simulink model "plant2016_cybership_non_adaptive"  (R2015b)
settings: Solver=VariableStepAuto  StartTime=0.0  StopTime=1000  RelTol=1e-3
libraries: simulink x4
settings Model: Creator=TordFO  LastModifiedBy=TordFO

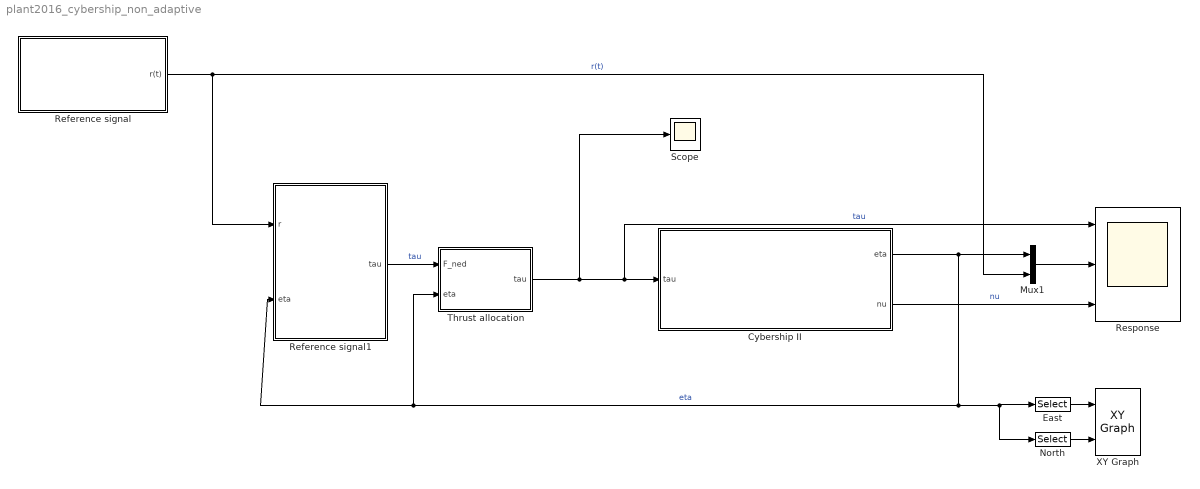
== system plant2016_cybership_non_adaptive ==
  Cybership II : Subsystem  mask{eta_0=[0;0;0]%[1;2;20*pi/180], nu_0=[0;0;0], first_order_waves_on_off=off, wind_on_off=on, surge_only=off}
      mask prompts: eta_0 "Position initial state"; nu_0 "Velocity initial state"; first_order_waves_on_off "First order wave disturbances"; wind_on_off "Wind loads"; surge_only "Only surge"
      mask Display: image('CybershipIII.jpg')
  East : Selector  InputPortWidth=3  IndexOptions=Index vector (dialog)  Indices=[2]  OutputSizes=1
  Mux1 : Mux  Inputs=2
  North : Selector  InputPortWidth=3  IndexOptions=Index vector (dialog)  Indices=[1]  OutputSizes=1
  Reference signal : Subsystem
  Reference signal1 : Subsystem  mask(SISO 3 DOF controller){surge_Kp=2.7, surge_Ki=0.1, surge_Kd=10, sway_Kp=2, sway_Ki=0.1, sway_Kd=10, yaw_Kp=2, yaw_Ki=0.3, yaw_Kd=2, surge_epsilon=0.01, sway_epsilon=0.01, yaw_epsilon=0.01}
      mask prompts: surge_Kp "Kp-gain"; surge_Ki "Ki-gain"; surge_Kd "Kd-gain"; sway_Kp "Kp-gain"; sway_Ki "Ki-gain"; sway_Kd "Kd-gain"; yaw_Kp "Kp-gain"; yaw_Ki "Ki-gain"; yaw_Kd "Kd-gain"; surge_epsilon "Surge epsilon"; sway_epsilon "Sway epsilon"; yaw_epsilon "Yaw epsilon"
      mask help: The masked subsystem is a 3 DOF controller for planear motion ship control. The controller replicates the structure of the self-tuning unfalsified PID controller, here with fixed gain to compare behaviour
      mask Help: Activate any combinations of the SISO controllers. Gains and epsolon values should be positive. Epsilon values are added derivative term in denominator to make controller biproper. Set gain values for activated controller other that zero (not required) to use the controller.
      mask Display: image('control_system.png')
  Response : Scope  NumInputPorts=3
  Scope : Scope
  Thrust allocation : Subsystem  mask(Thrust allocation block){surge_control_on_off=on, sway_control_on_off=on, yaw_control_on_off=on}
      mask prompts: surge_control_on_off "Surge Thrust on"; sway_control_on_off "Sway Thrust on"; yaw_control_on_off "Yaw Thrust on"
      mask help: Thrust allocation block. The block rotates the NED-force vector to the body frame where the ship is actuated in pure surge, sway and yaw. Any of the thrust direction can be enabeled/disabeled, but note that reference tracking is only possible for both surge and sway thrust enabeled.
  XY Graph : simulink/Sinks/XY Graph  xmin=-10  xmax=10  ymin=-10  ymax=10  st=-1
  wires:
  Reference signal/1(r(t)) -> Reference signal1/1(r), Mux1/2  "r(t)"
  Cybership II/2(nu) -> Response/3  "nu"
  Mux1/1 -> Response/2
  North/1 -> XY Graph/2
  East/1 -> XY Graph/1
  Cybership II/1(eta) -> Mux1/1, Reference signal1/2(eta), Thrust allocation/2(eta), North/1, East/1  "eta"
  Thrust allocation/1(tau) -> Scope/1, Cybership II/1(tau), Response/1  "tau"
  Reference signal1/1(tau) -> Thrust allocation/1(F_ned)  "tau"

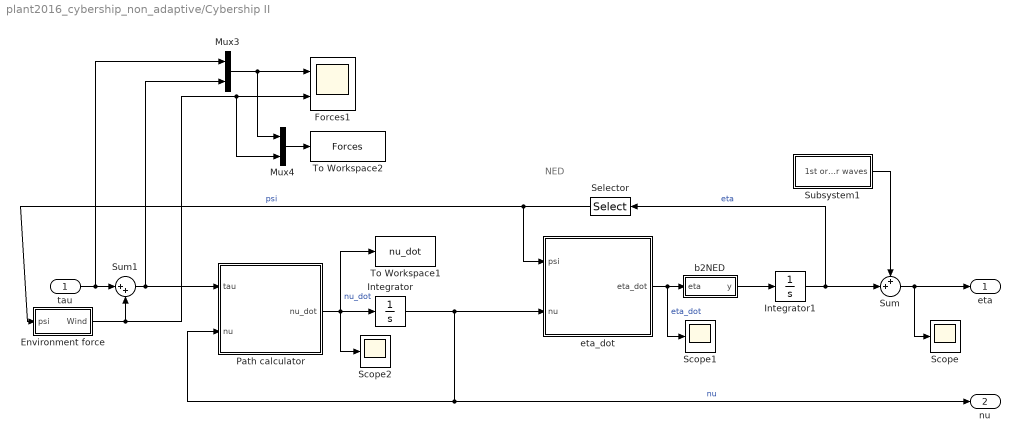
== system plant2016_cybership_non_adaptive/Cybership II ==
  note: NED
  tau : Inport
  Environment force : Subsystem
  Forces1 : Scope  NumInputPorts=2
  Integrator : Integrator  InitialCondition=nu_0
  Integrator1 : Integrator  InitialCondition=eta_0
  Mux3 : Mux  Inputs=2
  Mux4 : Mux  Inputs=2
  Path calculator : MATLAB Function  TreatAsAtomicUnit=on
  Scope : Scope
  Scope1 : Scope
  Scope2 : Scope
  Selector : Selector  InputPortWidth=3  IndexOptions=Index vector (dialog)  Indices=3  OutputSizes=1
  Subsystem1 : Subsystem
  Sum : Sum  Inputs=++|
  Sum1 : Sum  Inputs=|++
  To Workspace1 : ToWorkspace  VariableName=nu_dot  SaveFormat=Timeseries  SampleTime=-1
  To Workspace2 : ToWorkspace  VariableName=Forces  SaveFormat=Timeseries  SampleTime=-1
  b2NED : MATLAB Function  TreatAsAtomicUnit=on
  eta_dot : MATLAB Function  TreatAsAtomicUnit=on
  eta : Outport
  nu : Outport  Port=2
  wires:
  Sum1/1 -> Mux3/2, Path calculator/1(tau)
  eta_dot/1(eta_dot) -> Scope1/1, b2NED/1(eta)  "eta_dot"
  Path calculator/1(nu_dot) -> Scope2/1, To Workspace1/1, Integrator/1  "nu_dot"
  Integrator1/1 -> Sum/2, Selector/1  "eta"
  Integrator/1 -> nu/1, Path calculator/2(nu), eta_dot/2(nu)  "nu"
  Selector/1 -> eta_dot/1(psi), Environment force/1(psi)  "psi"
  b2NED/1(y) -> Integrator1/1
  Sum/1 -> Scope/1, eta/1
  Subsystem1/1(1st order waves) -> Sum/1
  tau/1 -> Mux3/1, Sum1/1
  Environment force/1(Wind) -> Forces1/2, Mux4/2, Sum1/2
  Mux3/1 -> Forces1/1, Mux4/1
  Mux4/1 -> To Workspace2/1

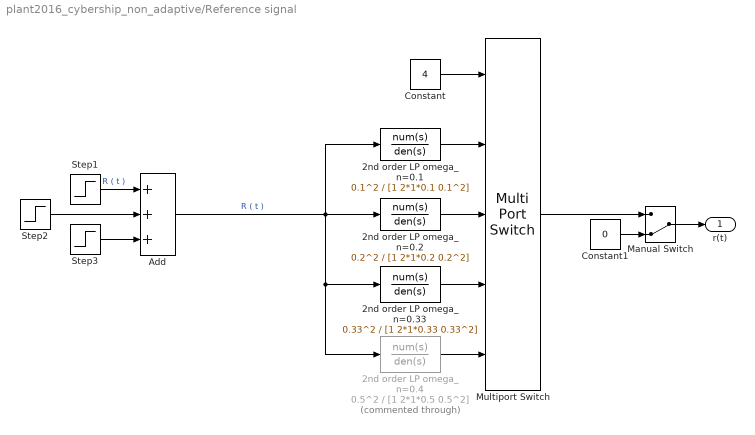
== system plant2016_cybership_non_adaptive/Reference signal ==
  2nd order LP omega_n=0.1 : TransferFcn  Numerator=0.1^2  Denominator=[1 2*1*0.1 0.1^2]
  2nd order LP omega_n=0.2 : TransferFcn  Numerator=0.2^2  Denominator=[1 2*1*0.2 0.2^2]
  2nd order LP omega_n=0.33 : TransferFcn  Numerator=0.33^2  Denominator=[1 2*1*0.33 0.33^2]
  2nd order LP omega_n=0.4 : TransferFcn  Commented=through  Numerator=0.5^2  Denominator=[1 2*1*0.5 0.5^2]
  Add : Sum  Inputs=+++
  Constant : Constant  Value=4
  Constant1 : Constant  Value=0
  Manual Switch : ManualSwitch  CurrentSetting=0
  Multiport Switch : MultiPortSwitch  Inputs=4
  Step1 : Step  Time=5  SampleTime=0
  Step2 : Step  Time=30  SampleTime=0
  Step3 : Step  Time=60  After=-2  SampleTime=0
  r(t) : Outport
  wires:
  Add/1 -> 2nd order LP omega_n=0.1/1, 2nd order LP omega_n=0.2/1, 2nd order LP omega_n=0.33/1, 2nd order LP omega_n=0.4/1  "R ( t )"
  Multiport Switch/1 -> Manual Switch/1
  2nd order LP omega_n=0.1/1 -> Multiport Switch/2
  2nd order LP omega_n=0.2/1 -> Multiport Switch/3
  2nd order LP omega_n=0.33/1 -> Multiport Switch/4
  Step1/1 -> Add/1  "R ( t )"
  Step2/1 -> Add/2
  Step3/1 -> Add/3
  2nd order LP omega_n=0.4/1 -> Multiport Switch/5
  Constant/1 -> Multiport Switch/1
  Manual Switch/1 -> r(t)/1
  Constant1/1 -> Manual Switch/2

== system plant2016_cybership_non_adaptive/Reference signal1 ==
  r : Inport
  eta : Inport  Port=2
  Demux : Demux  Outputs=3
  Mux : Mux  Inputs=3
  surge : Subsystem
  sway : Subsystem
  yaw : Subsystem
  tau : Outport
  wires:
  eta/1 -> Demux/1
  Demux/1 -> surge/2(eta_1)
  Demux/2 -> sway/2(eta_2)
  Demux/3 -> yaw/2(eta_3)
  surge/1(tau_1) -> Mux/1
  sway/1(tau_2) -> Mux/2
  yaw/1(tau_3) -> Mux/3
  r/1 -> surge/1(r), yaw/1(r), sway/1(r)
  Mux/1 -> tau/1

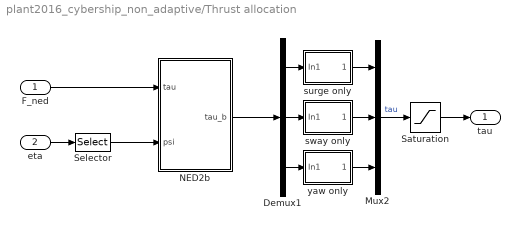
== system plant2016_cybership_non_adaptive/Thrust allocation ==
  F_ned : Inport
  eta : Inport  Port=2
  Demux1 : Demux  Outputs=3
  Mux2 : Mux  Inputs=3
  NED2b : MATLAB Function  TreatAsAtomicUnit=on
  Saturation : Saturate  UpperLimit=[10;10;10]  LowerLimit=[-10;-10;-10]
  Selector : Selector  InputPortWidth=3  IndexOptions=Index vector (dialog)  Indices=[3]  OutputSizes=1
  surge only : Subsystem
  sway only : Subsystem
  yaw only : Subsystem
  tau : Outport
  wires:
  Mux2/1 -> Saturation/1  "tau"
  Selector/1 -> NED2b/2(psi)
  F_ned/1 -> NED2b/1(tau)
  NED2b/1(tau_b) -> Demux1/1
  Demux1/3 -> yaw only/1(In1)
  yaw only/1(Out1) -> Mux2/3
  surge only/1(Out1) -> Mux2/1
  Demux1/2 -> sway only/1(In1)
  sway only/1(Out1) -> Mux2/2
  Demux1/1 -> surge only/1(In1)
  eta/1 -> Selector/1
  Saturation/1 -> tau/1

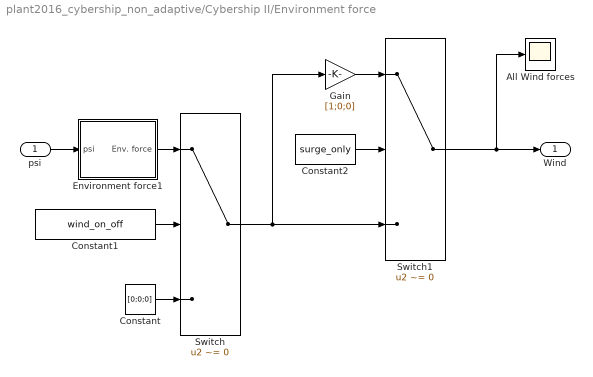
== system plant2016_cybership_non_adaptive/Cybership II/Environment force ==
  psi : Inport
  All Wind forces : Scope
  Constant : Constant  Value=[0;0;0]
  Constant1 : Constant  Value=wind_on_off
  Constant2 : Constant  Value=surge_only
  Environment force1 : Subsystem
  Gain : Gain  Gain=[1;0;0]
  Switch : Switch  Criteria=u2 ~= 0
  Switch1 : Switch  Criteria=u2 ~= 0
  Wind : Outport
  wires:
  psi/1 -> Environment force1/1(psi)
  Switch/1 -> Switch1/3, Gain/1
  Constant/1 -> Switch/3
  Constant1/1 -> Switch/2
  Environment force1/1(Env. force) -> Switch/1
  Switch1/1 -> Wind/1, All Wind forces/1
  Gain/1 -> Switch1/1
  Constant2/1 -> Switch1/2

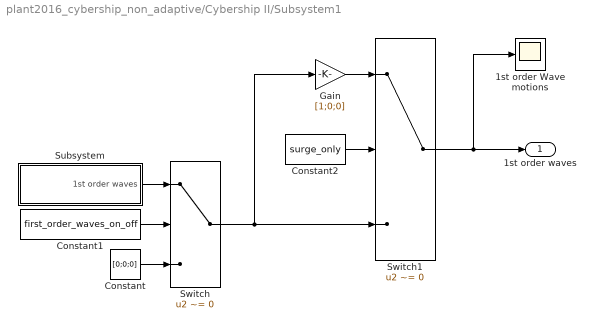
== system plant2016_cybership_non_adaptive/Cybership II/Subsystem1 ==
  1st order Wave motions : Scope
  Constant : Constant  Value=[0;0;0]
  Constant1 : Constant  Value=first_order_waves_on_off
  Constant2 : Constant  Value=surge_only
  Gain : Gain  Gain=[1;0;0]
  Subsystem : Subsystem  mask{start_time=0, omega_01=0.6, zeta_01=0.01, omega_02=0.6, zeta_02=0.1, omega_03=0.01, zeta_03=0.04}
      mask prompts: start_time "Wave start time"; omega_01 "Surge Dominating - wave frequency"; zeta_01 "Surge - Damping ratio"; omega_02 "Sway - Dominating wave frequency"; zeta_02 "Sway - Damping ratio"; omega_03 "Yaw - Dominating wave frequency"; zeta_03 "Yaw - Damping ratio"
      mask Display: disp('1st order Waves')
  Switch : Switch  Criteria=u2 ~= 0
  Switch1 : Switch  Criteria=u2 ~= 0
  1st order waves : Outport
  wires:
  Constant/1 -> Switch/3
  Constant1/1 -> Switch/2
  Subsystem/1(1st order waves) -> Switch/1
  Switch/1 -> Switch1/3, Gain/1
  Switch1/1 -> 1st order waves/1, 1st order Wave motions/1
  Gain/1 -> Switch1/1
  Constant2/1 -> Switch1/2

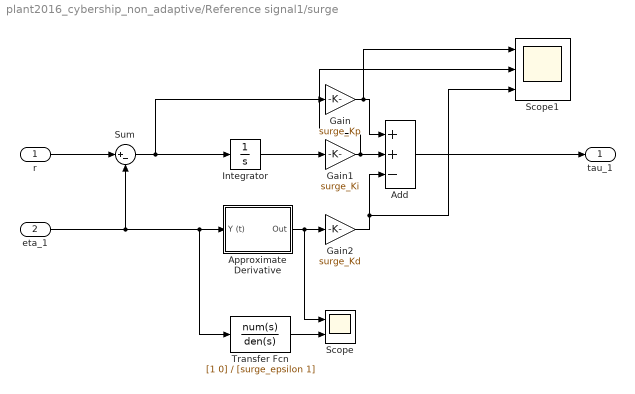
== system plant2016_cybership_non_adaptive/Reference signal1/surge ==
  r : Inport
  eta_1 : Inport  Port=2
  Add : Sum  Inputs=++-
  Approximate Derivative : Subsystem
  Gain : Gain  Gain=surge_Kp
  Gain1 : Gain  Gain=surge_Ki
  Gain2 : Gain  Gain=surge_Kd
  Integrator : Integrator
  Scope : Scope  NumInputPorts=2
  Scope1 : Scope  NumInputPorts=3
  Sum : Sum  Inputs=|+-
  Transfer Fcn : TransferFcn  Numerator=[1 0]  Denominator=[surge_epsilon 1]
  tau_1 : Outport
  wires:
  Sum/1 -> Integrator/1, Gain/1
  Gain2/1 -> Add/3, Scope1/3
  Integrator/1 -> Gain1/1
  Gain/1 -> Scope1/1, Add/1
  Approximate Derivative/1(Out) -> Scope/1, Gain2/1
  Add/1 -> tau_1/1
  eta_1/1 -> Sum/2, Transfer Fcn/1, Approximate Derivative/1(Y (t))
  Transfer Fcn/1 -> Scope/2
  r/1 -> Sum/1
  Gain1/1 -> Scope1/2, Add/2

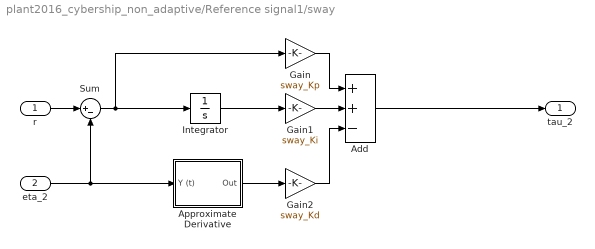
== system plant2016_cybership_non_adaptive/Reference signal1/sway ==
  r : Inport
  eta_2 : Inport  Port=2
  Add : Sum  Inputs=++-
  Approximate Derivative : Subsystem
  Gain : Gain  Gain=sway_Kp
  Gain1 : Gain  Gain=sway_Ki
  Gain2 : Gain  Gain=sway_Kd
  Integrator : Integrator
  Sum : Sum  Inputs=|+-
  tau_2 : Outport
  wires:
  Approximate Derivative/1(Out) -> Gain2/1
  Gain/1 -> Add/1
  Integrator/1 -> Gain1/1
  Gain2/1 -> Add/3
  Sum/1 -> Integrator/1, Gain/1
  Add/1 -> tau_2/1
  eta_2/1 -> Sum/2, Approximate Derivative/1(Y (t))
  Gain1/1 -> Add/2
  r/1 -> Sum/1

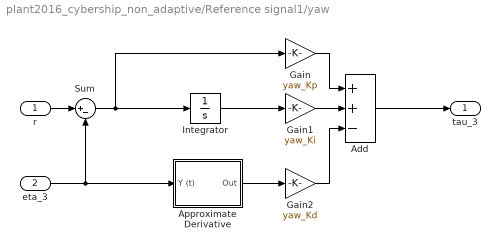
== system plant2016_cybership_non_adaptive/Reference signal1/yaw ==
  r : Inport
  eta_3 : Inport  Port=2
  Add : Sum  Inputs=++-
  Approximate Derivative : Subsystem
  Gain : Gain  Gain=yaw_Kp
  Gain1 : Gain  Gain=yaw_Ki
  Gain2 : Gain  Gain=yaw_Kd
  Integrator : Integrator
  Sum : Sum  Inputs=|+-
  tau_3 : Outport
  wires:
  Sum/1 -> Integrator/1, Gain/1
  Gain2/1 -> Add/3
  Integrator/1 -> Gain1/1
  Gain/1 -> Add/1
  Approximate Derivative/1(Out) -> Gain2/1
  Add/1 -> tau_3/1
  eta_3/1 -> Sum/2, Approximate Derivative/1(Y (t))
  Gain1/1 -> Add/2
  r/1 -> Sum/1

== system plant2016_cybership_non_adaptive/Thrust allocation/surge only ==
  In1 : Inport
  Constant : Constant  Value=0
  Constant1 : Constant  Value=surge_control_on_off
  Switch : Switch  Criteria=u2 ~= 0
  Out1 : Outport
  wires:
  Constant1/1 -> Switch/2
  Constant/1 -> Switch/3
  In1/1 -> Switch/1
  Switch/1 -> Out1/1

== system plant2016_cybership_non_adaptive/Thrust allocation/sway only ==
  In1 : Inport
  Constant2 : Constant  Value=0
  Constant3 : Constant  Value=sway_control_on_off
  Switch1 : Switch  Criteria=u2 ~= 0
  Out1 : Outport
  wires:
  In1/1 -> Switch1/1
  Switch1/1 -> Out1/1
  Constant3/1 -> Switch1/2
  Constant2/1 -> Switch1/3

== system plant2016_cybership_non_adaptive/Thrust allocation/yaw only ==
  In1 : Inport
  Constant : Constant  Value=0
  Constant1 : Constant  Value=yaw_control_on_off
  Switch : Switch  Criteria=u2 ~= 0
  Out1 : Outport
  wires:
  In1/1 -> Switch/1
  Switch/1 -> Out1/1
  Constant/1 -> Switch/3
  Constant1/1 -> Switch/2

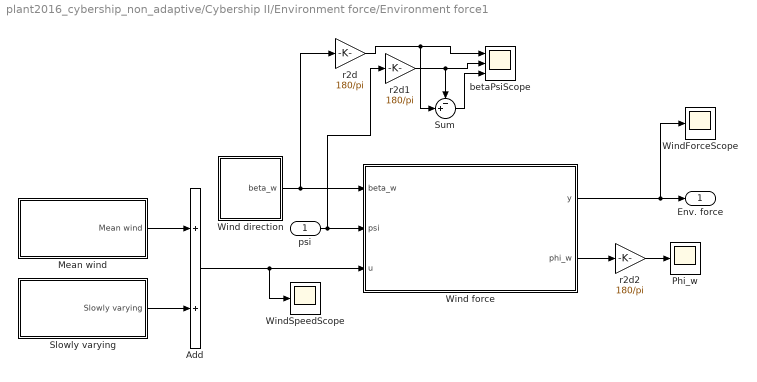
== system plant2016_cybership_non_adaptive/Cybership II/Environment force/Environment force1 ==
  psi : Inport
  Add : Sum  Inputs=2
  Mean wind : Subsystem  mask{windStrength=1, start=50}
      mask prompts: windStrength "Wind Strength"; start "Start Time"
  Phi_w : Scope
  Slowly varying : Subsystem  mask{start=70}
      mask prompts: start "Start Time"
  Sum : Sum  Inputs=-+|
  Wind direction : Subsystem
  Wind force : MATLAB Function  TreatAsAtomicUnit=on
  WindForceScope : Scope
  WindSpeedScope : Scope
  betaPsiScope : Scope  NumInputPorts=3
  r2d : Gain  Gain=180/pi
  r2d1 : Gain  Gain=180/pi
  r2d2 : Gain  Gain=180/pi
  Env. force : Outport
  wires:
  Add/1 -> WindSpeedScope/1, Wind force/3(u)
  Wind force/1(y) -> WindForceScope/1, Env. force/1
  psi/1 -> r2d1/1, Wind force/2(psi)
  Wind direction/1(beta_w) -> r2d/1, Wind force/1(beta_w)
  r2d/1 -> Sum/2, betaPsiScope/1
  Mean wind/1(Mean wind) -> Add/1
  Slowly varying/1(Slowly varying) -> Add/2
  r2d1/1 -> betaPsiScope/2, Sum/1
  Wind force/2(phi_w) -> r2d2/1
  r2d2/1 -> Phi_w/1
  Sum/1 -> betaPsiScope/3

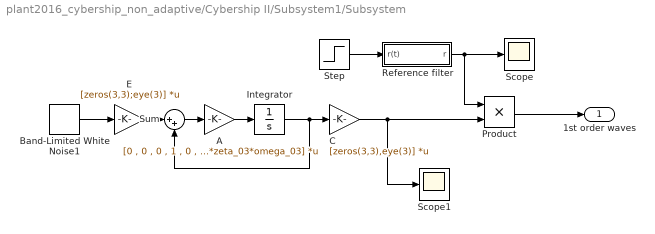
== system plant2016_cybership_non_adaptive/Cybership II/Subsystem1/Subsystem ==
  A : Gain  Gain=[0 , 0 , 0 , 1 , 0 , 0 ; 0 , 0 , 0 , 0 , 1 , 0 ; 0 , 0 , 0 , 0 , 0 , 1 ; -omega_01^2 , 0 , 0 , -2*zeta_01*omega_01 , 0 , 0 ; 0 ,- omega_02^2 , 0 , 0 , -2*zeta_02*omega_02 , 0 ; 0 , 0 , -omega_03^2 , 0 , 0 , -2*zeta_03*omega_03]  Multiplication=Matrix(K*u) (u vector)
  Band-Limited White Noise1 : simulink/Sources/Band-Limited White Noise  Cov=[0.01;0.01;0.01]  Ts=0.1  seed=[23341]
  C : Gain  Gain=[zeros(3,3),eye(3)]  Multiplication=Matrix(K*u) (u vector)
  E : Gain  Gain=[zeros(3,3);eye(3)]  Multiplication=Matrix(K*u) (u vector)
  Integrator : Integrator  InitialCondition=[0;0;0;0;0;0]
  Product : Product
  Reference filter : Subsystem  mask(2nd order lop pass filter){omega_0=0.4, zeta=1}
      mask prompts: omega_0 "Critical frequency"; zeta "Damping ratio"
      mask help: The masked subsystem is a 2nd order linear siso low-pass filter with parameters set in the edit boxes
      mask Display: disp('2nd order LP')
  Scope : Scope
  Scope1 : Scope
  Step : Step  Time=start_time  SampleTime=0
  Sum : Sum  Inputs=|++
  1st order waves : Outport
  wires:
  Band-Limited White Noise1/1 -> E/1
  A/1 -> Integrator/1
  Integrator/1 -> Sum/2, C/1
  Sum/1 -> A/1
  E/1 -> Sum/1
  C/1 -> Scope1/1, Product/2
  Step/1 -> Reference filter/1(r(t))
  Product/1 -> 1st order waves/1
  Reference filter/1(r) -> Scope/1, Product/1

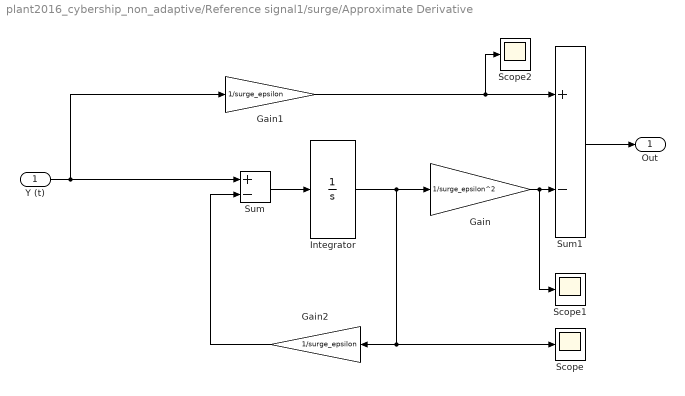
== system plant2016_cybership_non_adaptive/Reference signal1/surge/Approximate Derivative ==
  Y (t) : Inport
  Gain : Gain  Gain=1/surge_epsilon^2  SaturateOnIntegerOverflow=on  OutDataTypeStr=Inherit: Same as input  ParamDataTypeStr=Inherit: Same as input
  Gain1 : Gain  Gain=1/surge_epsilon  SaturateOnIntegerOverflow=on  OutDataTypeStr=Inherit: Same as input  ParamDataTypeStr=Inherit: Same as input
  Gain2 : Gain  Gain=1/surge_epsilon  SaturateOnIntegerOverflow=on  OutDataTypeStr=Inherit: Same as input  ParamDataTypeStr=Inherit: Same as input
  Integrator : Integrator
  Scope : Scope
  Scope1 : Scope
  Scope2 : Scope
  Sum : Sum  Inputs=+-  SaturateOnIntegerOverflow=on  InputSameDT=on  OutDataTypeStr=Inherit: Same as first input
  Sum1 : Sum  Inputs=+-  SaturateOnIntegerOverflow=on  InputSameDT=on  OutDataTypeStr=Inherit: Same as first input
  Out : Outport
  wires:
  Sum/1 -> Integrator/1
  Y (t)/1 -> Gain1/1, Sum/1
  Gain1/1 -> Scope2/1, Sum1/1
  Gain2/1 -> Sum/2
  Sum1/1 -> Out/1
  Gain/1 -> Scope1/1, Sum1/2
  Integrator/1 -> Gain2/1, Scope/1, Gain/1

== system plant2016_cybership_non_adaptive/Reference signal1/sway/Approximate Derivative ==
  Y (t) : Inport
  Gain : Gain  Gain=1/sway_epsilon^2  SaturateOnIntegerOverflow=on  OutDataTypeStr=Inherit: Same as input  ParamDataTypeStr=Inherit: Same as input
  Gain1 : Gain  Gain=1/sway_epsilon  SaturateOnIntegerOverflow=on  OutDataTypeStr=Inherit: Same as input  ParamDataTypeStr=Inherit: Same as input
  Gain2 : Gain  Gain=1/sway_epsilon  SaturateOnIntegerOverflow=on  OutDataTypeStr=Inherit: Same as input  ParamDataTypeStr=Inherit: Same as input
  Integrator : Integrator
  Sum : Sum  Inputs=+-  SaturateOnIntegerOverflow=on  InputSameDT=on  OutDataTypeStr=Inherit: Same as first input
  Sum1 : Sum  Inputs=+-  SaturateOnIntegerOverflow=on  InputSameDT=on  OutDataTypeStr=Inherit: Same as first input
  Out : Outport
  wires:
  Integrator/1 -> Gain/1, Gain2/1
  Gain/1 -> Sum1/2
  Sum1/1 -> Out/1
  Gain2/1 -> Sum/2
  Gain1/1 -> Sum1/1
  Y (t)/1 -> Sum/1, Gain1/1
  Sum/1 -> Integrator/1

== system plant2016_cybership_non_adaptive/Reference signal1/yaw/Approximate Derivative ==
  Y (t) : Inport
  Gain : Gain  Gain=1/yaw_epsilon^2  SaturateOnIntegerOverflow=on  OutDataTypeStr=Inherit: Same as input  ParamDataTypeStr=Inherit: Same as input
  Gain1 : Gain  Gain=1/yaw_epsilon  SaturateOnIntegerOverflow=on  OutDataTypeStr=Inherit: Same as input  ParamDataTypeStr=Inherit: Same as input
  Gain2 : Gain  Gain=1/yaw_epsilon  SaturateOnIntegerOverflow=on  OutDataTypeStr=Inherit: Same as input  ParamDataTypeStr=Inherit: Same as input
  Integrator : Integrator
  Sum : Sum  Inputs=+-  SaturateOnIntegerOverflow=on  InputSameDT=on  OutDataTypeStr=Inherit: Same as first input
  Sum1 : Sum  Inputs=+-  SaturateOnIntegerOverflow=on  InputSameDT=on  OutDataTypeStr=Inherit: Same as first input
  Out : Outport
  wires:
  Sum/1 -> Integrator/1
  Y (t)/1 -> Gain1/1, Sum/1
  Gain1/1 -> Sum1/1
  Gain2/1 -> Sum/2
  Sum1/1 -> Out/1
  Gain/1 -> Sum1/2
  Integrator/1 -> Gain2/1, Gain/1

== system plant2016_cybership_non_adaptive/Cybership II/Environment force/Environment force1/Mean wind ==
  Constant4 : Constant  Value=windStrength
  Product : Product
  Reference filter : Subsystem
  Start1 : Step  Time=start  SampleTime=0
  Mean wind : Outport
  wires:
  Constant4/1 -> Product/2
  Start1/1 -> Product/1
  Reference filter/1(r) -> Mean wind/1  "mean_wind"
  Product/1 -> Reference filter/1(r(t))

== system plant2016_cybership_non_adaptive/Cybership II/Environment force/Environment force1/Slowly varying ==
  1st order Markov2 : Subsystem
  Band-Limited White Noise1 : simulink/Sources/Band-Limited White Noise  Cov=1  Ts=0.1  seed=[23341]
  Product : Product
  Reference filter : Subsystem
  Scope : Scope
  Start1 : Step  Time=100  SampleTime=0
  Slowly varying : Outport
  wires:
  Product/1 -> Reference filter/1(r(t))  "Slowly"
  Start1/1 -> Product/1
  1st order Markov2/1(Out1) -> Product/2
  Band-Limited White Noise1/1 -> 1st order Markov2/1(In1)
  Reference filter/1(r) -> Scope/1, Slowly varying/1

== system plant2016_cybership_non_adaptive/Cybership II/Environment force/Environment force1/Wind direction ==
  note: OBS: beta_w \in [0,360)
  1st order Markov2 : Subsystem
  Band-Limited White Noise1 : simulink/Sources/Band-Limited White Noise  Cov=10  Ts=0.1  seed=[23341]
  beta_w : Outport
  wires:
  1st order Markov2/1(Out1) -> beta_w/1
  Band-Limited White Noise1/1 -> 1st order Markov2/1(In1)

== system plant2016_cybership_non_adaptive/Cybership II/Subsystem1/Subsystem/Reference filter ==
  r(t) : Inport
  2nd order LP1 : TransferFcn  Numerator=omega_0^2  Denominator=[1 2*zeta*omega_0 omega_0^2]
  r : Outport
  wires:
  r(t)/1 -> 2nd order LP1/1
  2nd order LP1/1 -> r/1

== system plant2016_cybership_non_adaptive/Cybership II/Environment force/Environment force1/Mean wind/Reference filter ==
  r(t) : Inport
  2nd order LP1 : TransferFcn  Numerator=0.3^2  Denominator=[1 2*1*0.3 0.3^2]
  r : Outport
  wires:
  r(t)/1 -> 2nd order LP1/1
  2nd order LP1/1 -> r/1

== system plant2016_cybership_non_adaptive/Cybership II/Environment force/Environment force1/Slowly varying/1st order Markov2 ==
  In1 : Inport
  Gain : Gain  Gain=2
  Sum : Sum  Inputs=|+-
  Transfer Fcn : TransferFcn  Denominator=[50 1]
  Out1 : Outport
  wires:
  In1/1 -> Sum/1
  Sum/1 -> Transfer Fcn/1
  Transfer Fcn/1 -> Sum/2, Gain/1
  Gain/1 -> Out1/1

== system plant2016_cybership_non_adaptive/Cybership II/Environment force/Environment force1/Slowly varying/Reference filter ==
  r(t) : Inport
  2nd order LP1 : TransferFcn  Numerator=0.1^2  Denominator=[1 2*1*0.1 0.1^2]
  r : Outport
  wires:
  r(t)/1 -> 2nd order LP1/1
  2nd order LP1/1 -> r/1

== system plant2016_cybership_non_adaptive/Cybership II/Environment force/Environment force1/Wind direction/1st order Markov2 ==
  In1 : Inport
  2nd order LP1 : TransferFcn  Numerator=0.005^2  Denominator=[1 2*1*0.005 0.005^2]
  Constant : Constant  Value=2*pi*rand()
  Constant1 : Constant  Commented=on  Value=30*pi/180 + pi
  Gain : Gain  Gain=2
  Sum : Sum  Inputs=|+-
  Sum1 : Sum  Inputs=++|
  Out1 : Outport
  wires:
  In1/1 -> Sum/1
  Sum/1 -> 2nd order LP1/1
  2nd order LP1/1 -> Gain/1
  Constant/1 -> Sum1/1
  Gain/1 -> Sum1/2, Sum/2
  Sum1/1 -> Out1/1

== matlab function plant2016_cybership_non_adaptive/Thrust allocation/NED2b ==
  data: tau input; tau_b output size=3; psi input
function tau_b = fcn(tau,psi)
R = [   cos(psi)    -sin(psi)   0
        sin(psi)     cos(psi)   0
        0            0          1];
tau_b = R'*tau;

== matlab function plant2016_cybership_non_adaptive/Cybership II/Path calculator ==
  data: tau input; nu input; nu_dot output
function nu_dot = fcn(tau,nu)
%% Cybership I
% % % m = 14.79;
% % % Iz = 1.76;
% % % xg = 0.0375;
% % % yg = 0;
% % % 
% % % Xudot   = -2;
% % % Yvdot   = -10;
% % % Yrdot   = 0;
% % % Nrdot   = -1;
% % % 
% % % Xu      = -0.4543;
% % % Yv      = -3.083;
% % % Yr      = -7.25;
% % % Nv      = 4.1117e-4;
% % % Nr      = -1.9;
% % % 
% % % M = [m-Xudot 0 0
% % %     0 m-Yvdot m*xg-Yrdot
% % %     0 m*xg - Yrdot Iz-Nrdot];
% % % 
% % % 
% % % D = [-Xu 0 0
% % %     0 -Yv -Yr    
% % %     0 -Nv -Nr];
% % % 
% % % nu_dot = -M\D*nu + M\tau;


%% Cybership II
% Data taken from: 
% @article{RN768,
%    author = {Hassani, Vahid and Pascoal, António M. and Aguiar, A. Pedro and Athans, Michael},
%    title = {A Multiple Model Adaptive Wave Filter for Dynamic Ship Positioning},
%    journal = {IFAC Proceedings Volumes},
%    volume = {43},
%    number = {20},
%    pages = {120-125},
%    ISSN = {1474-6670},
%    DOI = {http://dx.doi.org/10.3182/20100915-3-DE-3008.00026},
%    url = {http://www.sciencedirect.com/science/article/pii/S1474667016334486},
%    year = {2010},
%    type = {Journal Article}
% }


M = [   25.8,       0,          0;
        0,          33.8,       1.0115;
        0,          1.0115,     2.76];
    
D = [   2,          0,          0;
        0,          7,          0.1;
        0,          0.1,        0.5];

nu_dot = -M\D*nu + M\tau;

end

== matlab function plant2016_cybership_non_adaptive/Cybership II/eta_dot ==
  data: psi input; nu input; eta_dot output
function eta_dot = fcn(psi,nu)

R = [   cos(psi)    -sin(psi)   0
        sin(psi)     cos(psi)   0
        0            0          1];

eta_dot = R*nu;

end

== matlab function plant2016_cybership_non_adaptive/Cybership II/Environment force/Environment force1/Wind force ==
  data: beta_w input; psi input; u input; y output; phi_w output
function [y,phi_w] = fcn(beta_w,psi,u)
CX = 0.70;  % CX \in {0.50,0.90}
CY = 0.87;  % CY \in {0.70,0.95}
CN = 0.05;  % CN \in {0.05,0.20} - After reccomodations found on p.191 in Fossen

phi_w = rad2pipi(beta_w-psi);

R = [  -CX*cos(phi_w);
       -CY*sin(phi_w);
       -CN*sin(2*phi_w)];

y = u.*R;

== matlab function plant2016_cybership_non_adaptive/Cybership II/b2NED ==
  data: eta input; y output
function y = rad2pipi(eta)

angle = eta(3);
r = rem(angle+sign(angle)*pi,2*pi);
s = sign(sign(angle) + 2*(sign(abs(rem(angle+pi,2*pi)/(2*pi)))-1));

y = [   eta(1);
        eta(2);
        r - s*pi];
